simulink model "boat_sim_ss_bruce"  (R2018b)
settings: Solver=VariableStepAuto  StartTime=0.0  StopTime=20  RelTol=1e-3
undefined symbols (not defined in the file or in its folder): linearized_B_disturb, state_eq
(part 2 of 2)

== matlab function boat_sim_ss_bruce/non_linear_plant/MATLAB Function ==
  data: x input; alpha_tw input; x_dot output size=1; phi input; psi input; rangle input; roll input; sangle input; surge input; sway input; v_tw input; yaw input; y_dot output size=1; phi_dot output size=1; psi_dot output size=1; surge_dot output size=1; sway_dot output size=1; roll_dot output size=1; yaw_dot output size=1
function [x_dot, y_dot, phi_dot, psi_dot, surge_dot, sway_dot, roll_dot, yaw_dot]=get_states_dot(x,alpha_tw, phi, psi, rangle, roll, sangle, surge, sway, v_tw, yaw)
% alpha_tw=1; phi=1; psi=1; rangle=1; roll=1; sangle=1; surge=1; sway=1; v_tw=1; yaw=1;

function Y = heaviside(X)
%HEAVISIDE    Step function.
Y = zeros(size(X));
Y(X > 0) = 1;
Y(X == 0) = .5;
end

output =[
 
                                                                                                                                                                                                                                                                                                                                                                                                                                                                                                                                                                                                                                                                                                                                                                                                                                                                                                                                                                                                                                                                                                                                                                                                                                                                                                                                                                                                                                                                                                                                                                                                                                                                                                                                                                                                                                                                                                                                                                                                                                                                                                                                                                                                                                                                                                                                                                                                                                                                                                                                                                                                                                                                                                                                                                                                                                                                                                                                                                                                                                                                                                                                                                                                                                                                                                                                                                                                                                                                                                                                                                                                                                                                                                                                                                                                                                                                                                                                                                                                                                                                                                                                                                                                                                                                                                                                                                                                                                                                                                                                                                                                                                                                                                                                                                                                                                                                                                                                                                                                                                                                                                                                                                                                                                                                                                                                                                                                                                                                                                                                                                                                                                                                                                                                                                                                                                                                                                                                                                                                                                                                                                                                                                                                                                                                                                                                                                               surge*cos(psi) - sway*cos(phi)*sin(psi)
                                                                                                                                                                                                                                                                                                                                                                                                                                                                                                                                                                                                                                                                                                                                                                                                                                                                                                                                                                                                                                                                                                                                                                                                                                                                                                                                                                                                                                                                                                                                                                                                                                                                                                                                                                                                                                                                                                                                                                                                                                                                                                                                                                                                                                                                                                                                                                                                                                                                                                                                                                                                                                                                                                                                                                                                                                                                                                                                                                                                                                                                                                                                                                                                                                                                                                                                                                                                                                                                                                                                                                                                                                                                                                                                                                                                                                                                                                                                                                                                                                                                                                                                                                                                                                                                                                                                                                                                                                                                                                                                                                                                                                                                                                                                                                                                                                                                                                                                                                                                                                                                                                                                                                                                                                                                                                                                                                                                                                                                                                                                                                                                                                                                                                                                                                                                                                                                                                                                                                                                                                                                                                                                                                                                                                                                                                                                                                               surge*sin(psi) + sway*cos(phi)*cos(psi)
                                                                                                                                                                                                                                                                                                                                                                                                                                                                                                                                                                                                                                                                                                                                                                                                                                                                                                                                                                                                                                                                                                                                                                                                                                                                                                                                                                                                                                                                                                                                                                                                                                                                                                                                                                                                                                                                                                                                                                                                                                                                                                                                                                                                                                                                                                                                                                                                                                                                                                                                                                                                                                                                                                                                                                                                                                                                                                                                                                                                                                                                                                                                                                                                                                                                                                                                                                                                                                                                                                                                                                                                                                                                                                                                                                                                                                                                                                                                                                                                                                                                                                                                                                                                                                                                                                                                                                                                                                                                                                                                                                                                                                                                                                                                                                                                                                                                                                                                                                                                                                                                                                                                                                                                                                                                                                                                                                                                                                                                                                                                                                                                                                                                                                                                                                                                                                                                                                                                                                                                                                                                                                                                                                                                                                                                                                                                                                                                                  roll
                                                                                                                                                                                                                                                                                                                                                                                                                                                                                                                                                                                                                                                                                                                                                                                                                                                                                                                                                                                                                                                                                                                                                                                                                                                                                                                                                                                                                                                                                                                                                                                                                                                                                                                                                                                                                                                                                                                                                                                                                                                                                                                                                                                                                                                                                                                                                                                                                                                                                                                                                                                                                                                                                                                                                                                                                                                                                                                                                                                                                                                                                                                                                                                                                                                                                                                                                                                                                                                                                                                                                                                                                                                                                                                                                                                                                                                                                                                                                                                                                                                                                                                                                                                                                                                                                                                                                                                                                                                                                                                                                                                                                                                                                                                                                                                                                                                                                                                                                                                                                                                                                                                                                                                                                                                                                                                                                                                                                                                                                                                                                                                                                                                                                                                                                                                                                                                                                                                                                                                                                                                                                                                                                                                                                                                                                                                                                                                                          yaw*cos(phi)
                                                                                                                                                                                                                                                                                                                                                                                                                                                                                                                                                                                                                                                                                                                                                                                                                                                                                                                                                                                                                                                                                                                                                                                                                                                                                                                                                                                                                                                                                                                                                                                                                                                                                                                                                                                                                                                                                                                                                                                                                                                                                                                                                                                                                                                                                                                                                                                                                                                                                                                                                                                                                                                                                                                    (997*yaw)/1997 - (1000*sway*yaw)/1997 + (997*(abs(surge - yaw)^2 + abs(sway - roll + yaw)^2/abs(cos(phi))^2)*(cos(2*rangle - 2*angle((surge - yaw/10)/(abs(surge - yaw/10)^2 + abs(sway - (3*roll)/10 + yaw/10)^2)^(1/2) - ((sway - (3*roll)/10 + yaw/10)*1i)/(abs(surge - yaw/10)^2 + abs(sway - (3*roll)/10 + yaw/10)^2)^(1/2))) - 1))/3994 + (997*(imag((sway - roll + yaw)/(cos(phi)*(abs(surge - yaw)^2 + abs(sway - roll + yaw)^2/abs(cos(phi))^2)^(1/2))) + (real(surge) - real(yaw))/(abs(surge - yaw)^2 + abs(sway - roll + yaw)^2/abs(cos(phi))^2)^(1/2))*(cos(2*angle((surge - yaw)/(abs(surge - yaw)^2 + abs(sway - roll + yaw)^2/abs(cos(phi))^2)^(1/2) - ((sway - roll + yaw)*1i)/(cos(phi)*(abs(surge - yaw)^2 + abs(sway - roll + yaw)^2/abs(cos(phi))^2)^(1/2)))) - 1)*(abs(surge - yaw)^2 + abs(sway - roll + yaw)^2/abs(cos(phi))^2))/(3994*abs((surge - yaw)/(abs(surge - yaw)^2 + abs(sway - roll + yaw)^2/abs(cos(phi))^2)^(1/2) - ((sway - roll + yaw)*1i)/(cos(phi)*(abs(surge - yaw)^2 + abs(sway - roll + yaw)^2/abs(cos(phi))^2)^(1/2)))) + (332775788538406563*sin(2*sangle - 2*angle(((3*roll - sway + yaw + v_tw*sin(alpha_tw - psi)*cos(phi))*1i)/(abs(yaw - surge + v_tw*cos(alpha_tw - psi))^2 + abs(3*roll - sway + yaw + v_tw*sin(alpha_tw - psi)*cos(phi))^2)^(1/2) - (yaw - surge + v_tw*cos(alpha_tw - psi))/(abs(yaw - surge + v_tw*cos(alpha_tw - psi))^2 + abs(3*roll - sway + yaw + v_tw*sin(alpha_tw - psi)*cos(phi))^2)^(1/2)))*(abs(yaw - surge + v_tw*cos(alpha_tw - psi))^2 + abs(3*roll - sway + yaw + v_tw*sin(alpha_tw - psi)*cos(phi))^2)*((imag(v_tw*cos(alpha_tw - psi)) - imag(surge) + imag(yaw))/(abs(yaw - surge + v_tw*cos(alpha_tw - psi))^2 + abs(3*roll - sway + yaw + v_tw*sin(alpha_tw - psi)*cos(phi))^2)^(1/2) - (real(v_tw*sin(alpha_tw - psi)*cos(phi)) + 3*real(roll) - real(sway) + real(yaw))/(abs(yaw - surge + v_tw*cos(alpha_tw - psi))^2 + abs(3*roll - sway + yaw + v_tw*sin(alpha_tw - psi)*cos(phi))^2)^(1/2)))/(89936884558588805120*abs((yaw - surge + v_tw*cos(alpha_tw - psi))/(abs(yaw - surge + v_tw*cos(alpha_tw - psi))^2 + abs(3*roll - sway + yaw + v_tw*sin(alpha_tw - psi)*cos(phi))^2)^(1/2) - ((3*roll - sway + yaw + v_tw*sin(alpha_tw - psi)*cos(phi))*1i)/(abs(yaw - surge + v_tw*cos(alpha_tw - psi))^2 + abs(3*roll - sway + yaw + v_tw*sin(alpha_tw - psi)*cos(phi))^2)^(1/2))) - (332775788538406563*(cos(2*sangle - 2*angle(((3*roll - sway + yaw + v_tw*sin(alpha_tw - psi)*cos(phi))*1i)/(abs(yaw - surge + v_tw*cos(alpha_tw - psi))^2 + abs(3*roll - sway + yaw + v_tw*sin(alpha_tw - psi)*cos(phi))^2)^(1/2) - (yaw - surge + v_tw*cos(alpha_tw - psi))/(abs(yaw - surge + v_tw*cos(alpha_tw - psi))^2 + abs(3*roll - sway + yaw + v_tw*sin(alpha_tw - psi)*cos(phi))^2)^(1/2))) - 1)*(abs(yaw - surge + v_tw*cos(alpha_tw - psi))^2 + abs(3*roll - sway + yaw + v_tw*sin(alpha_tw - psi)*cos(phi))^2)*((3*imag(roll) - imag(sway) + imag(yaw) + imag(v_tw*sin(alpha_tw - psi)*cos(phi)))/(abs(yaw - surge + v_tw*cos(alpha_tw - psi))^2 + abs(3*roll - sway + yaw + v_tw*sin(alpha_tw - psi)*cos(phi))^2)^(1/2) + (real(v_tw*cos(alpha_tw - psi)) - real(surge) + real(yaw))/(abs(yaw - surge + v_tw*cos(alpha_tw - psi))^2 + abs(3*roll - sway + yaw + v_tw*sin(alpha_tw - psi)*cos(phi))^2)^(1/2)))/(89936884558588805120*abs((yaw - surge + v_tw*cos(alpha_tw - psi))/(abs(yaw - surge + v_tw*cos(alpha_tw - psi))^2 + abs(3*roll - sway + yaw + v_tw*sin(alpha_tw - psi)*cos(phi))^2)^(1/2) - ((3*roll - sway + yaw + v_tw*sin(alpha_tw - psi)*cos(phi))*1i)/(abs(yaw - surge + v_tw*cos(alpha_tw - psi))^2 + abs(3*roll - sway + yaw + v_tw*sin(alpha_tw - psi)*cos(phi))^2)^(1/2)))
                                                                                                                                                                                                                                                                                                                                                                                                                                                                                                                                                                                                                                                                                                                                                                                                                                                                                                                                                                                                                                                                                                                                                                                                                                                                                                                                                                                                                                                                                                                                                                                                                                                                                                                                                                                                                                                                                                                                                                                                                                                                                                                                                                                                                                                                                                                                                                                                                                                                                                                                                                                                                                                                                                                   (1000*surge*yaw)/1997 - (997*yaw)/1997 - (997*sin(2*rangle - 2*angle((surge - yaw/10)/(abs(surge - yaw/10)^2 + abs(sway - (3*roll)/10 + yaw/10)^2)^(1/2) - ((sway - (3*roll)/10 + yaw/10)*1i)/(abs(surge - yaw/10)^2 + abs(sway - (3*roll)/10 + yaw/10)^2)^(1/2)))*(abs(sway - (3*roll)/10 + yaw/10)^2 + abs(surge - yaw/10)^2))/3994 + (332775788538406563*(cos(2*sangle - 2*angle(((3*roll - sway + yaw + v_tw*sin(alpha_tw - psi)*cos(phi))*1i)/(abs(yaw - surge + v_tw*cos(alpha_tw - psi))^2 + abs(3*roll - sway + yaw + v_tw*sin(alpha_tw - psi)*cos(phi))^2)^(1/2) - (yaw - surge + v_tw*cos(alpha_tw - psi))/(abs(yaw - surge + v_tw*cos(alpha_tw - psi))^2 + abs(3*roll - sway + yaw + v_tw*sin(alpha_tw - psi)*cos(phi))^2)^(1/2))) - 1)*(abs(yaw - surge + v_tw*cos(alpha_tw - psi))^2 + abs(3*roll - sway + yaw + v_tw*sin(alpha_tw - psi)*cos(phi))^2)*((imag(v_tw*cos(alpha_tw - psi)) - imag(surge) + imag(yaw))/(abs(yaw - surge + v_tw*cos(alpha_tw - psi))^2 + abs(3*roll - sway + yaw + v_tw*sin(alpha_tw - psi)*cos(phi))^2)^(1/2) - (real(v_tw*sin(alpha_tw - psi)*cos(phi)) + 3*real(roll) - real(sway) + real(yaw))/(abs(yaw - surge + v_tw*cos(alpha_tw - psi))^2 + abs(3*roll - sway + yaw + v_tw*sin(alpha_tw - psi)*cos(phi))^2)^(1/2)))/(89936884558588805120*abs((yaw - surge + v_tw*cos(alpha_tw - psi))/(abs(yaw - surge + v_tw*cos(alpha_tw - psi))^2 + abs(3*roll - sway + yaw + v_tw*sin(alpha_tw - psi)*cos(phi))^2)^(1/2) - ((3*roll - sway + yaw + v_tw*sin(alpha_tw - psi)*cos(phi))*1i)/(abs(yaw - surge + v_tw*cos(alpha_tw - psi))^2 + abs(3*roll - sway + yaw + v_tw*sin(alpha_tw - psi)*cos(phi))^2)^(1/2))) + (332775788538406563*sin(2*sangle - 2*angle(((3*roll - sway + yaw + v_tw*sin(alpha_tw - psi)*cos(phi))*1i)/(abs(yaw - surge + v_tw*cos(alpha_tw - psi))^2 + abs(3*roll - sway + yaw + v_tw*sin(alpha_tw - psi)*cos(phi))^2)^(1/2) - (yaw - surge + v_tw*cos(alpha_tw - psi))/(abs(yaw - surge + v_tw*cos(alpha_tw - psi))^2 + abs(3*roll - sway + yaw + v_tw*sin(alpha_tw - psi)*cos(phi))^2)^(1/2)))*(abs(yaw - surge + v_tw*cos(alpha_tw - psi))^2 + abs(3*roll - sway + yaw + v_tw*sin(alpha_tw - psi)*cos(phi))^2)*((3*imag(roll) - imag(sway) + imag(yaw) + imag(v_tw*sin(alpha_tw - psi)*cos(phi)))/(abs(yaw - surge + v_tw*cos(alpha_tw - psi))^2 + abs(3*roll - sway + yaw + v_tw*sin(alpha_tw - psi)*cos(phi))^2)^(1/2) + (real(v_tw*cos(alpha_tw - psi)) - real(surge) + real(yaw))/(abs(yaw - surge + v_tw*cos(alpha_tw - psi))^2 + abs(3*roll - sway + yaw + v_tw*sin(alpha_tw - psi)*cos(phi))^2)^(1/2)))/(89936884558588805120*abs((yaw - surge + v_tw*cos(alpha_tw - psi))/(abs(yaw - surge + v_tw*cos(alpha_tw - psi))^2 + abs(3*roll - sway + yaw + v_tw*sin(alpha_tw - psi)*cos(phi))^2)^(1/2) - ((3*roll - sway + yaw + v_tw*sin(alpha_tw - psi)*cos(phi))*1i)/(abs(yaw - surge + v_tw*cos(alpha_tw - psi))^2 + abs(3*roll - sway + yaw + v_tw*sin(alpha_tw - psi)*cos(phi))^2)^(1/2))) + (997*cos(phi)*(cos(2*angle((surge - yaw)/(abs(surge - yaw)^2 + abs(sway - roll + yaw)^2/abs(cos(phi))^2)^(1/2) - ((sway - roll + yaw)*1i)/(cos(phi)*(abs(surge - yaw)^2 + abs(sway - roll + yaw)^2/abs(cos(phi))^2)^(1/2)))) - 1)*(abs(surge - yaw)^2 + abs(sway - roll + yaw)^2/abs(cos(phi))^2)*(real((sway - roll + yaw)/(cos(phi)*(abs(surge - yaw)^2 + abs(sway - roll + yaw)^2/abs(cos(phi))^2)^(1/2))) - (imag(surge) - imag(yaw))/(abs(surge - yaw)^2 + abs(sway - roll + yaw)^2/abs(cos(phi))^2)^(1/2)))/(3994*abs((surge - yaw)/(abs(surge - yaw)^2 + abs(sway - roll + yaw)^2/abs(cos(phi))^2)^(1/2) - ((sway - roll + yaw)*1i)/(cos(phi)*(abs(surge - yaw)^2 + abs(sway - roll + yaw)^2/abs(cos(phi))^2)^(1/2))))
                                                                                                                                                                                                                                                                                                                                                                                                                                                                                                                                                                                                                                                                                                                                                                                                                                                                                                                                                                                                                                                                                                                                                                                                                                                                                                                                                                                                                                                                                                                                                                                                                                                                                                                                                                                                                                                                                                                                                                                                                                                                                                                                                                     (heaviside(x)*((6556092342678323*x)/68719476736 - (6556092342678323*pi)/68719476736 + (97827*cos(x))/5 + 99987*sin(x) - (3071362037134131*(x - pi)^2)/137438953472 - (3801231599547187*(x - pi)^3)/137438953472 - (2125075601025925*(x - pi)^4)/549755813888 + 19651))/1097 + (heaviside(-x)*((6556092342678323*x)/68719476736 + (6556092342678323*pi)/68719476736 - (97827*cos(x))/5 + 99987*sin(x) + (3071362037134131*(x + pi)^2)/137438953472 - (3801231599547187*(x + pi)^3)/137438953472 + (2125075601025925*(x + pi)^4)/549755813888 - 19651))/1097 - (roll*abs(roll))/1097 - (2991*sin(2*rangle - 2*angle((surge - yaw/10)/(abs(surge - yaw/10)^2 + abs(sway - (3*roll)/10 + yaw/10)^2)^(1/2) - ((sway - (3*roll)/10 + yaw/10)*1i)/(abs(surge - yaw/10)^2 + abs(sway - (3*roll)/10 + yaw/10)^2)^(1/2)))*(abs(sway - (3*roll)/10 + yaw/10)^2 + abs(surge - yaw/10)^2))/21940 + (998327365615219689*(cos(2*sangle - 2*angle(((3*roll - sway + yaw + v_tw*sin(alpha_tw - psi)*cos(phi))*1i)/(abs(yaw - surge + v_tw*cos(alpha_tw - psi))^2 + abs(3*roll - sway + yaw + v_tw*sin(alpha_tw - psi)*cos(phi))^2)^(1/2) - (yaw - surge + v_tw*cos(alpha_tw - psi))/(abs(yaw - surge + v_tw*cos(alpha_tw - psi))^2 + abs(3*roll - sway + yaw + v_tw*sin(alpha_tw - psi)*cos(phi))^2)^(1/2))) - 1)*(abs(yaw - surge + v_tw*cos(alpha_tw - psi))^2 + abs(3*roll - sway + yaw + v_tw*sin(alpha_tw - psi)*cos(phi))^2)*((imag(v_tw*cos(alpha_tw - psi)) - imag(surge) + imag(yaw))/(abs(yaw - surge + v_tw*cos(alpha_tw - psi))^2 + abs(3*roll - sway + yaw + v_tw*sin(alpha_tw - psi)*cos(phi))^2)^(1/2) - (real(v_tw*sin(alpha_tw - psi)*cos(phi)) + 3*real(roll) - real(sway) + real(yaw))/(abs(yaw - surge + v_tw*cos(alpha_tw - psi))^2 + abs(3*roll - sway + yaw + v_tw*sin(alpha_tw - psi)*cos(phi))^2)^(1/2)))/(49404487912254341120*abs((yaw - surge + v_tw*cos(alpha_tw - psi))/(abs(yaw - surge + v_tw*cos(alpha_tw - psi))^2 + abs(3*roll - sway + yaw + v_tw*sin(alpha_tw - psi)*cos(phi))^2)^(1/2) - ((3*roll - sway + yaw + v_tw*sin(alpha_tw - psi)*cos(phi))*1i)/(abs(yaw - surge + v_tw*cos(alpha_tw - psi))^2 + abs(3*roll - sway + yaw + v_tw*sin(alpha_tw - psi)*cos(phi))^2)^(1/2))) + (998327365615219689*sin(2*sangle - 2*angle(((3*roll - sway + yaw + v_tw*sin(alpha_tw - psi)*cos(phi))*1i)/(abs(yaw - surge + v_tw*cos(alpha_tw - psi))^2 + abs(3*roll - sway + yaw + v_tw*sin(alpha_tw - psi)*cos(phi))^2)^(1/2) - (yaw - surge + v_tw*cos(alpha_tw - psi))/(abs(yaw - surge + v_tw*cos(alpha_tw - psi))^2 + abs(3*roll - sway + yaw + v_tw*sin(alpha_tw - psi)*cos(phi))^2)^(1/2)))*(abs(yaw - surge + v_tw*cos(alpha_tw - psi))^2 + abs(3*roll - sway + yaw + v_tw*sin(alpha_tw - psi)*cos(phi))^2)*((3*imag(roll) - imag(sway) + imag(yaw) + imag(v_tw*sin(alpha_tw - psi)*cos(phi)))/(abs(yaw - surge + v_tw*cos(alpha_tw - psi))^2 + abs(3*roll - sway + yaw + v_tw*sin(alpha_tw - psi)*cos(phi))^2)^(1/2) + (real(v_tw*cos(alpha_tw - psi)) - real(surge) + real(yaw))/(abs(yaw - surge + v_tw*cos(alpha_tw - psi))^2 + abs(3*roll - sway + yaw + v_tw*sin(alpha_tw - psi)*cos(phi))^2)^(1/2)))/(49404487912254341120*abs((yaw - surge + v_tw*cos(alpha_tw - psi))/(abs(yaw - surge + v_tw*cos(alpha_tw - psi))^2 + abs(3*roll - sway + yaw + v_tw*sin(alpha_tw - psi)*cos(phi))^2)^(1/2) - ((3*roll - sway + yaw + v_tw*sin(alpha_tw - psi)*cos(phi))*1i)/(abs(yaw - surge + v_tw*cos(alpha_tw - psi))^2 + abs(3*roll - sway + yaw + v_tw*sin(alpha_tw - psi)*cos(phi))^2)^(1/2))) + (997*cos(phi)*(cos(2*angle((surge - yaw)/(abs(surge - yaw)^2 + abs(sway - roll + yaw)^2/abs(cos(phi))^2)^(1/2) - ((sway - roll + yaw)*1i)/(cos(phi)*(abs(surge - yaw)^2 + abs(sway - roll + yaw)^2/abs(cos(phi))^2)^(1/2)))) - 1)*(abs(surge - yaw)^2 + abs(sway - roll + yaw)^2/abs(cos(phi))^2)*(real((sway - roll + yaw)/(cos(phi)*(abs(surge - yaw)^2 + abs(sway - roll + yaw)^2/abs(cos(phi))^2)^(1/2))) - (imag(surge) - imag(yaw))/(abs(surge - yaw)^2 + abs(sway - roll + yaw)^2/abs(cos(phi))^2)^(1/2)))/(2194*abs((surge - yaw)/(abs(surge - yaw)^2 + abs(sway - roll + yaw)^2/abs(cos(phi))^2)^(1/2) - ((sway - roll + yaw)*1i)/(cos(phi)*(abs(surge - yaw)^2 + abs(sway - roll + yaw)^2/abs(cos(phi))^2)^(1/2))))
 (997*sway)/1097 - (997*surge)/1097 - (((332775788538406563*(cos(2*sangle - 2*angle(((3*roll - sway + yaw + v_tw*sin(alpha_tw - psi)*cos(phi))*1i)/(abs(yaw - surge + v_tw*cos(alpha_tw - psi))^2 + abs(3*roll - sway + yaw + v_tw*sin(alpha_tw - psi)*cos(phi))^2)^(1/2) - (yaw - surge + v_tw*cos(alpha_tw - psi))/(abs(yaw - surge + v_tw*cos(alpha_tw - psi))^2 + abs(3*roll - sway + yaw + v_tw*sin(alpha_tw - psi)*cos(phi))^2)^(1/2))) - 1)*(abs(yaw - surge + v_tw*cos(alpha_tw - psi))^2 + abs(3*roll - sway + yaw + v_tw*sin(alpha_tw - psi)*cos(phi))^2)*((imag(v_tw*cos(alpha_tw - psi)) - imag(surge) + imag(yaw))/(abs(yaw - surge + v_tw*cos(alpha_tw - psi))^2 + abs(3*roll - sway + yaw + v_tw*sin(alpha_tw - psi)*cos(phi))^2)^(1/2) - (real(v_tw*sin(alpha_tw - psi)*cos(phi)) + 3*real(roll) - real(sway) + real(yaw))/(abs(yaw - surge + v_tw*cos(alpha_tw - psi))^2 + abs(3*roll - sway + yaw + v_tw*sin(alpha_tw - psi)*cos(phi))^2)^(1/2)))/(45035996273704960*abs((yaw - surge + v_tw*cos(alpha_tw - psi))/(abs(yaw - surge + v_tw*cos(alpha_tw - psi))^2 + abs(3*roll - sway + yaw + v_tw*sin(alpha_tw - psi)*cos(phi))^2)^(1/2) - ((3*roll - sway + yaw + v_tw*sin(alpha_tw - psi)*cos(phi))*1i)/(abs(yaw - surge + v_tw*cos(alpha_tw - psi))^2 + abs(3*roll - sway + yaw + v_tw*sin(alpha_tw - psi)*cos(phi))^2)^(1/2))) + (332775788538406563*sin(2*sangle - 2*angle(((3*roll - sway + yaw + v_tw*sin(alpha_tw - psi)*cos(phi))*1i)/(abs(yaw - surge + v_tw*cos(alpha_tw - psi))^2 + abs(3*roll - sway + yaw + v_tw*sin(alpha_tw - psi)*cos(phi))^2)^(1/2) - (yaw - surge + v_tw*cos(alpha_tw - psi))/(abs(yaw - surge + v_tw*cos(alpha_tw - psi))^2 + abs(3*roll - sway + yaw + v_tw*sin(alpha_tw - psi)*cos(phi))^2)^(1/2)))*(abs(yaw - surge + v_tw*cos(alpha_tw - psi))^2 + abs(3*roll - sway + yaw + v_tw*sin(alpha_tw - psi)*cos(phi))^2)*((3*imag(roll) - imag(sway) + imag(yaw) + imag(v_tw*sin(alpha_tw - psi)*cos(phi)))/(abs(yaw - surge + v_tw*cos(alpha_tw - psi))^2 + abs(3*roll - sway + yaw + v_tw*sin(alpha_tw - psi)*cos(phi))^2)^(1/2) + (real(v_tw*cos(alpha_tw - psi)) - real(surge) + real(yaw))/(abs(yaw - surge + v_tw*cos(alpha_tw - psi))^2 + abs(3*roll - sway + yaw + v_tw*sin(alpha_tw - psi)*cos(phi))^2)^(1/2)))/(45035996273704960*abs((yaw - surge + v_tw*cos(alpha_tw - psi))/(abs(yaw - surge + v_tw*cos(alpha_tw - psi))^2 + abs(3*roll - sway + yaw + v_tw*sin(alpha_tw - psi)*cos(phi))^2)^(1/2) - ((3*roll - sway + yaw + v_tw*sin(alpha_tw - psi)*cos(phi))*1i)/(abs(yaw - surge + v_tw*cos(alpha_tw - psi))^2 + abs(3*roll - sway + yaw + v_tw*sin(alpha_tw - psi)*cos(phi))^2)^(1/2))))*(11^(1/2)*cos(sangle) - 1/2))/1097 + (997*sin(2*rangle - 2*angle((surge - yaw/10)/(abs(surge - yaw/10)^2 + abs(sway - (3*roll)/10 + yaw/10)^2)^(1/2) - ((sway - (3*roll)/10 + yaw/10)*1i)/(abs(surge - yaw/10)^2 + abs(sway - (3*roll)/10 + yaw/10)^2)^(1/2)))*(abs(sway - (3*roll)/10 + yaw/10)^2 + abs(surge - yaw/10)^2))/21940 - (yaw*cos(phi)*abs(yaw))/1097 - (11^(1/2)*sin(sangle)*((332775788538406563*sin(2*sangle - 2*angle(((3*roll - sway + yaw + v_tw*sin(alpha_tw - psi)*cos(phi))*1i)/(abs(yaw - surge + v_tw*cos(alpha_tw - psi))^2 + abs(3*roll - sway + yaw + v_tw*sin(alpha_tw - psi)*cos(phi))^2)^(1/2) - (yaw - surge + v_tw*cos(alpha_tw - psi))/(abs(yaw - surge + v_tw*cos(alpha_tw - psi))^2 + abs(3*roll - sway + yaw + v_tw*sin(alpha_tw - psi)*cos(phi))^2)^(1/2)))*(abs(yaw - surge + v_tw*cos(alpha_tw - psi))^2 + abs(3*roll - sway + yaw + v_tw*sin(alpha_tw - psi)*cos(phi))^2)*((imag(v_tw*cos(alpha_tw - psi)) - imag(surge) + imag(yaw))/(abs(yaw - surge + v_tw*cos(alpha_tw - psi))^2 + abs(3*roll - sway + yaw + v_tw*sin(alpha_tw - psi)*cos(phi))^2)^(1/2) - (real(v_tw*sin(alpha_tw - psi)*cos(phi)) + 3*real(roll) - real(sway) + real(yaw))/(abs(yaw - surge + v_tw*cos(alpha_tw - psi))^2 + abs(3*roll - sway + yaw + v_tw*sin(alpha_tw - psi)*cos(phi))^2)^(1/2)))/(45035996273704960*abs((yaw - surge + v_tw*cos(alpha_tw - psi))/(abs(yaw - surge + v_tw*cos(alpha_tw - psi))^2 + abs(3*roll - sway + yaw + v_tw*sin(alpha_tw - psi)*cos(phi))^2)^(1/2) - ((3*roll - sway + yaw + v_tw*sin(alpha_tw - psi)*cos(phi))*1i)/(abs(yaw - surge + v_tw*cos(alpha_tw - psi))^2 + abs(3*roll - sway + yaw + v_tw*sin(alpha_tw - psi)*cos(phi))^2)^(1/2))) - (332775788538406563*(cos(2*sangle - 2*angle(((3*roll - sway + yaw + v_tw*sin(alpha_tw - psi)*cos(phi))*1i)/(abs(yaw - surge + v_tw*cos(alpha_tw - psi))^2 + abs(3*roll - sway + yaw + v_tw*sin(alpha_tw - psi)*cos(phi))^2)^(1/2) - (yaw - surge + v_tw*cos(alpha_tw - psi))/(abs(yaw - surge + v_tw*cos(alpha_tw - psi))^2 + abs(3*roll - sway + yaw + v_tw*sin(alpha_tw - psi)*cos(phi))^2)^(1/2))) - 1)*(abs(yaw - surge + v_tw*cos(alpha_tw - psi))^2 + abs(3*roll - sway + yaw + v_tw*sin(alpha_tw - psi)*cos(phi))^2)*((3*imag(roll) - imag(sway) + imag(yaw) + imag(v_tw*sin(alpha_tw - psi)*cos(phi)))/(abs(yaw - surge + v_tw*cos(alpha_tw - psi))^2 + abs(3*roll - sway + yaw + v_tw*sin(alpha_tw - psi)*cos(phi))^2)^(1/2) + (real(v_tw*cos(alpha_tw - psi)) - real(surge) + real(yaw))/(abs(yaw - surge + v_tw*cos(alpha_tw - psi))^2 + abs(3*roll - sway + yaw + v_tw*sin(alpha_tw - psi)*cos(phi))^2)^(1/2)))/(45035996273704960*abs((yaw - surge + v_tw*cos(alpha_tw - psi))/(abs(yaw - surge + v_tw*cos(alpha_tw - psi))^2 + abs(3*roll - sway + yaw + v_tw*sin(alpha_tw - psi)*cos(phi))^2)^(1/2) - ((3*roll - sway + yaw + v_tw*sin(alpha_tw - psi)*cos(phi))*1i)/(abs(yaw - surge + v_tw*cos(alpha_tw - psi))^2 + abs(3*roll - sway + yaw + v_tw*sin(alpha_tw - psi)*cos(phi))^2)^(1/2)))))/1097 - (997*cos(phi)*(cos(2*angle((surge - yaw)/(abs(surge - yaw)^2 + abs(sway - roll + yaw)^2/abs(cos(phi))^2)^(1/2) - ((sway - roll + yaw)*1i)/(cos(phi)*(abs(surge - yaw)^2 + abs(sway - roll + yaw)^2/abs(cos(phi))^2)^(1/2)))) - 1)*(abs(surge - yaw)^2 + abs(sway - roll + yaw)^2/abs(cos(phi))^2)*(real((sway - roll + yaw)/(cos(phi)*(abs(surge - yaw)^2 + abs(sway - roll + yaw)^2/abs(cos(phi))^2)^(1/2))) - (imag(surge) - imag(yaw))/(abs(surge - yaw)^2 + abs(sway - roll + yaw)^2/abs(cos(phi))^2)^(1/2)))/(2194*abs((surge - yaw)/(abs(surge - yaw)^2 + abs(sway - roll + yaw)^2/abs(cos(phi))^2)^(1/2) - ((sway - roll + yaw)*1i)/(cos(phi)*(abs(surge - yaw)^2 + abs(sway - roll + yaw)^2/abs(cos(phi))^2)^(1/2))))
]
x_dot=output(1);
    y_dot =output(2);
    phi_dot=output(3); 
    psi_dot=output(4);
    surge_dot=output(5);
    sway_dot=output(6);
    roll_dot=output(7);
    yaw_dot=output(8);

end
